simulink model "SkywalkerX8_Lateral_Control"  (R2018a)
settings: Solver=FixedStepAuto  StartTime=0.0  StopTime=inf  FixedStep=0.001  RelTol=1e-3
undefined symbols (not defined in the file): SkywalkerX8
libraries: simulink_extras x1
settings Model: EnablePacing=on  Creator=David  LastModifiedBy=David

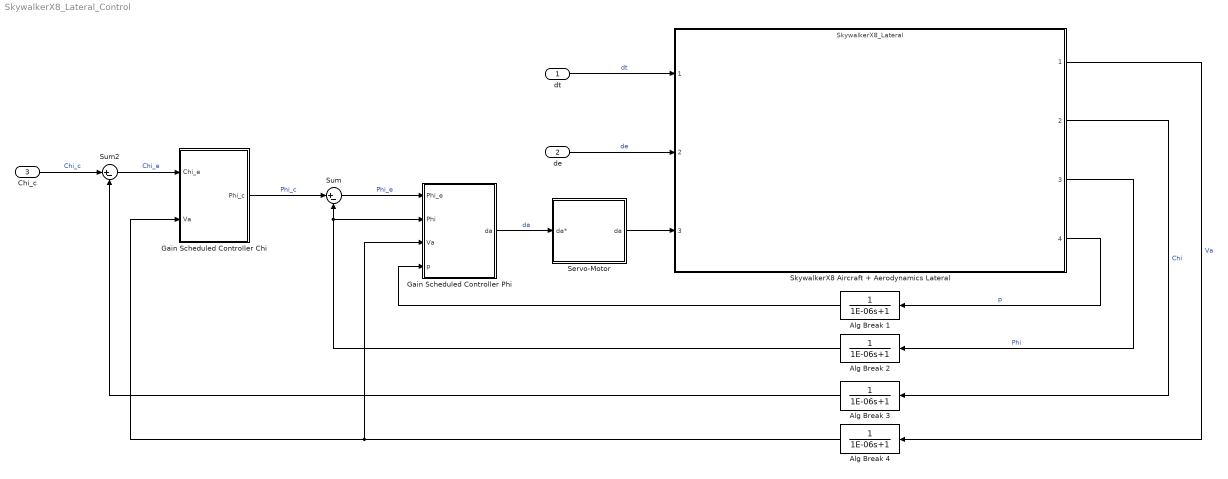
== system SkywalkerX8_Lateral_Control ==
  dt : Inport
  de : Inport  Port=2
  Chi_c : Inport  Port=3
  Alg Break {1..4} (4 alike) : TransferFcn  Denominator=[1E-06 1]
  Gain Scheduled Controller Chi : Subsystem
  Gain Scheduled Controller Phi : Subsystem
  Servo-Motor : Subsystem
      mask Display: image('servo.jpg', 'center')
  SkywalkerX8 Aircraft + Aerodynamics Lateral : ModelReference  ModelNameDialog=SkywalkerX8_Lateral.slx  ModelReferenceVersion=1.51
      mask Display:
      | image('x8SkySunset.png', 'center')
      | 
      | port_label('input', 1, '\delta_t (Unitless)', 'texmode', 'on')
      | port_label('input', 2, '\delta_e (rad)', 'texmode', 'on')
      | port_label('input', 3, '\delta_a (rad)', 'texmode', 'on')
      | 
      | port_label('output', 1, 'V_a (m/s)', 'texmode', 'on')
      | port_label('output', 2, '\chi (rad)', 'texmode', 'on')
      | port_label('output', 3, '\Phi (rad)', 'texmode', 'on')
      | port_label('output', 4, 'p (rad/s)', 'texmode', 'on')
  Sum : Sum  Inputs=|+-
  Sum2 : Sum  Inputs=|+-
  wires:
  SkywalkerX8 Aircraft + Aerodynamics Lateral/3 -> Alg Break 2/1  "Phi"
  SkywalkerX8 Aircraft + Aerodynamics Lateral/1 -> Alg Break 4/1  "Va"
  SkywalkerX8 Aircraft + Aerodynamics Lateral/2 -> Alg Break 3/1  "Chi"
  Gain Scheduled Controller Chi/1(Phi_c) -> Sum/1  "Phi_c"
  Chi_c/1 -> Sum2/1  "Chi_c"
  Sum/1 -> Gain Scheduled Controller Phi/1(Phi_e)  "Phi_e"
  Sum2/1 -> Gain Scheduled Controller Chi/1(Chi_e)  "Chi_e"
  Alg Break 4/1 -> Gain Scheduled Controller Chi/2(Va), Gain Scheduled Controller Phi/3(Va)
  Alg Break 2/1 -> Gain Scheduled Controller Phi/2(Phi), Sum/2
  Gain Scheduled Controller Phi/1(da) -> Servo-Motor/1(da*)  "da"
  Alg Break 1/1 -> Gain Scheduled Controller Phi/4(p)
  de/1 -> SkywalkerX8 Aircraft + Aerodynamics Lateral/2  "de"
  dt/1 -> SkywalkerX8 Aircraft + Aerodynamics Lateral/1  "dt"
  SkywalkerX8 Aircraft + Aerodynamics Lateral/4 -> Alg Break 1/1  "p"
  Alg Break 3/1 -> Sum2/2
  Servo-Motor/1(da) -> SkywalkerX8 Aircraft + Aerodynamics Lateral/3

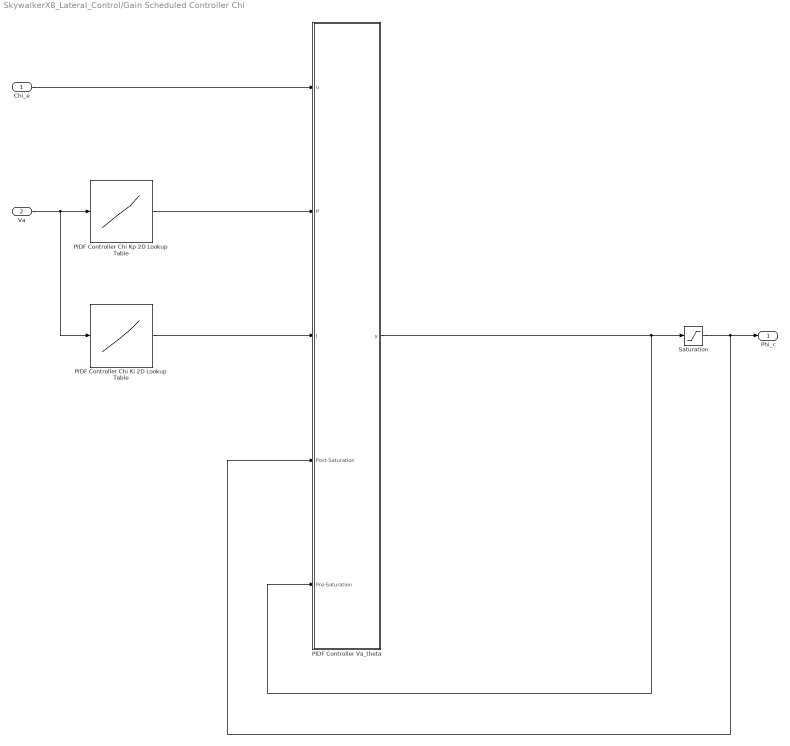
== system SkywalkerX8_Lateral_Control/Gain Scheduled Controller Chi ==
  Chi_e : Inport
  Va : Inport  Port=2
  PIDF Controller Chi Ki 2D Lookup Table : Lookup_n-D  NumberOfTableDimensions=1  BreakpointsForDimension1=SkywalkerX8.Control.Lateral.SchedulingVariables.VaArray  BreakpointsForDimension2=SkywalkerX8.Control.Longitudinal.SchedulingVariables.alphaArray  Table=SkywalkerX8.Control.Lateral.ChiController.KiChi  InternalRulePriority=Speed  RndMeth=Simplest  InputSameDT=on
  PIDF Controller Chi Kp 2D Lookup Table : Lookup_n-D  NumberOfTableDimensions=1  BreakpointsForDimension1=SkywalkerX8.Control.Lateral.SchedulingVariables.VaArray  BreakpointsForDimension2=SkywalkerX8.Control.Longitudinal.SchedulingVariables.alphaArray  Table=SkywalkerX8.Control.Lateral.ChiController.KpChi  InternalRulePriority=Speed  RndMeth=Simplest  InputSameDT=on
  PIDF Controller Va_theta : Subsystem
  Saturation : Saturate  UpperLimit=SkywalkerX8.Control.Lateral.ChiController.upperSaturationPhiC  LowerLimit=SkywalkerX8.Control.Lateral.ChiController.lowerSaturationPhiC
  Phi_c : Outport
  wires:
  PIDF Controller Chi Kp 2D Lookup Table/1 -> PIDF Controller Va_theta/2(P)
  Chi_e/1 -> PIDF Controller Va_theta/1(u)
  Va/1 -> PIDF Controller Chi Ki 2D Lookup Table/1, PIDF Controller Chi Kp 2D Lookup Table/1
  PIDF Controller Chi Ki 2D Lookup Table/1 -> PIDF Controller Va_theta/3(I)
  Saturation/1 -> PIDF Controller Va_theta/4(Post-Saturation), Phi_c/1
  PIDF Controller Va_theta/1(y) -> PIDF Controller Va_theta/5(Pre-Saturation), Saturation/1

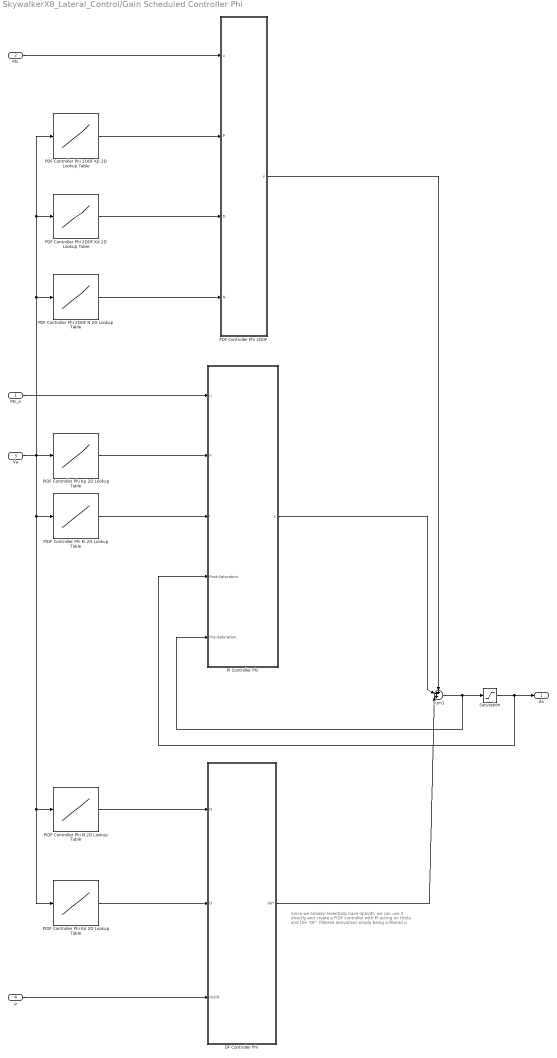
== system SkywalkerX8_Lateral_Control/Gain Scheduled Controller Phi ==
  note: Since we already essentially have dphi/dt,
      | we can use it directly and create a PIDF controller
      | with PI acting on theta and the "DF" (filtered derivative)
      | simply being a filtered p
  Phi_e : Inport
  Phi : Inport  Port=2
  Va : Inport  Port=3
  p : Inport  Port=4
  DF Controller Phi : Subsystem
  PDF Controller Phi 2DOF : Subsystem
  PDF Controller Phi 2DOF Kd 2D Lookup Table : Lookup_n-D  NumberOfTableDimensions=1  BreakpointsForDimension1=SkywalkerX8.Control.Lateral.SchedulingVariables.VaArray  BreakpointsForDimension2=SkywalkerX8.Control.Longitudinal.SchedulingVariables.alphaArray  Table=SkywalkerX8.Control.Lateral.PhiController.KdPhi2DOF  InternalRulePriority=Speed  RndMeth=Simplest  InputSameDT=on
  PDF Controller Phi 2DOF Kp 2D Lookup Table : Lookup_n-D  NumberOfTableDimensions=1  BreakpointsForDimension1=SkywalkerX8.Control.Lateral.SchedulingVariables.VaArray  BreakpointsForDimension2=SkywalkerX8.Control.Longitudinal.SchedulingVariables.alphaArray  Table=SkywalkerX8.Control.Lateral.PhiController.KpPhi2DOF  InternalRulePriority=Speed  RndMeth=Simplest  InputSameDT=on
  PDF Controller Phi 2DOF N 2D Lookup Table : Lookup_n-D  NumberOfTableDimensions=1  BreakpointsForDimension1=SkywalkerX8.Control.Lateral.SchedulingVariables.VaArray  BreakpointsForDimension2=SkywalkerX8.Control.Longitudinal.SchedulingVariables.alphaArray  Table=SkywalkerX8.Control.Lateral.PhiController.NPhi2DOF  InternalRulePriority=Speed  RndMeth=Simplest  InputSameDT=on
  PI Controller Phi : Subsystem
  PIDF Controller Phi Kd 2D Lookup Table : Lookup_n-D  NumberOfTableDimensions=1  BreakpointsForDimension1=SkywalkerX8.Control.Lateral.SchedulingVariables.VaArray  BreakpointsForDimension2=SkywalkerX8.Control.Longitudinal.SchedulingVariables.alphaArray  Table=SkywalkerX8.Control.Lateral.PhiController.KdPhi  InternalRulePriority=Speed  RndMeth=Simplest  InputSameDT=on
  PIDF Controller Phi Ki 2D Lookup Table : Lookup_n-D  NumberOfTableDimensions=1  BreakpointsForDimension1=SkywalkerX8.Control.Lateral.SchedulingVariables.VaArray  BreakpointsForDimension2=SkywalkerX8.Control.Longitudinal.SchedulingVariables.alphaArray  Table=SkywalkerX8.Control.Lateral.PhiController.KiPhi  InternalRulePriority=Speed  RndMeth=Simplest  InputSameDT=on
  PIDF Controller Phi Kp 2D Lookup Table : Lookup_n-D  NumberOfTableDimensions=1  BreakpointsForDimension1=SkywalkerX8.Control.Lateral.SchedulingVariables.VaArray  BreakpointsForDimension2=SkywalkerX8.Control.Longitudinal.SchedulingVariables.alphaArray  Table=SkywalkerX8.Control.Lateral.PhiController.KpPhi  InternalRulePriority=Speed  RndMeth=Simplest  InputSameDT=on
  PIDF Controller Phi N 2D Lookup Table : Lookup_n-D  NumberOfTableDimensions=1  BreakpointsForDimension1=SkywalkerX8.Control.Lateral.SchedulingVariables.VaArray  BreakpointsForDimension2=SkywalkerX8.Control.Longitudinal.SchedulingVariables.alphaArray  Table=SkywalkerX8.Control.Lateral.PhiController.NPhi  InternalRulePriority=Speed  RndMeth=Simplest  InputSameDT=on
  Saturation : Saturate  UpperLimit=SkywalkerX8.Control.Lateral.PhiController.upperSaturationDa  LowerLimit=SkywalkerX8.Control.Lateral.PhiController.lowerSaturationDa
  Sum1 : Sum  Inputs=+++|
  da : Outport
  wires:
  Va/1 -> PDF Controller Phi 2DOF Kp 2D Lookup Table/1, PDF Controller Phi 2DOF Kd 2D Lookup Table/1, PDF Controller Phi 2DOF N 2D Lookup Table/1, PIDF Controller Phi N 2D Lookup Table/1, PIDF Controller Phi Kd 2D Lookup Table/1, PIDF Controller Phi Ki 2D Lookup Table/1, PIDF Controller Phi Kp 2D Lookup Table/1
  Phi_e/1 -> PI Controller Phi/1(u)
  PIDF Controller Phi Kp 2D Lookup Table/1 -> PI Controller Phi/2(P)
  PIDF Controller Phi Ki 2D Lookup Table/1 -> PI Controller Phi/3(I)
  PI Controller Phi/1(y) -> Sum1/2
  Sum1/1 -> Saturation/1, PI Controller Phi/5(Pre-Saturation)
  p/1 -> DF Controller Phi/3(du/dt)
  DF Controller Phi/1(da*) -> Sum1/3
  PIDF Controller Phi N 2D Lookup Table/1 -> DF Controller Phi/1(N)
  PIDF Controller Phi Kd 2D Lookup Table/1 -> DF Controller Phi/2(D)
  Saturation/1 -> da/1, PI Controller Phi/4(Post-Saturation)
  PDF Controller Phi 2DOF Kp 2D Lookup Table/1 -> PDF Controller Phi 2DOF/2(P)
  PDF Controller Phi 2DOF Kd 2D Lookup Table/1 -> PDF Controller Phi 2DOF/3(D)
  PDF Controller Phi 2DOF N 2D Lookup Table/1 -> PDF Controller Phi 2DOF/4(N)
  Phi/1 -> PDF Controller Phi 2DOF/1(u)
  PDF Controller Phi 2DOF/1(y) -> Sum1/1

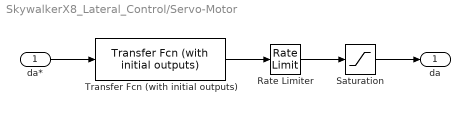
== system SkywalkerX8_Lateral_Control/Servo-Motor ==
  da* : Inport
  Rate Limiter : RateLimiter  RisingSlewLimit=SkywalkerX8.Actuators.Servos.RateLimit  FallingSlewLimit=-SkywalkerX8.Actuators.Servos.RateLimit  SampleTimeMode=inherited  InitialCondition=SkywalkerX8.InitialConditions.de
  Saturation : Saturate  UpperLimit=2*SkywalkerX8.Actuators.Servos.UpperSaturation  LowerLimit=2*SkywalkerX8.Actuators.Servos.LowerSaturation
  Transfer Fcn (with initial outputs) : simulink_extras/Additional Linear/Transfer Fcn (with initial outputs)  N=cell2mat(SkywalkerX8.Actuators.Servos.TF.Numerator)  D=cell2mat(SkywalkerX8.Actuators.Servos.TF.Denominator)  Y0=SkywalkerX8.InitialConditions.da  U0=SkywalkerX8.InitialConditions.da
  da : Outport
  wires:
  Rate Limiter/1 -> Saturation/1
  da*/1 -> Transfer Fcn (with initial outputs)/1
  Saturation/1 -> da/1
  Transfer Fcn (with initial outputs)/1 -> Rate Limiter/1

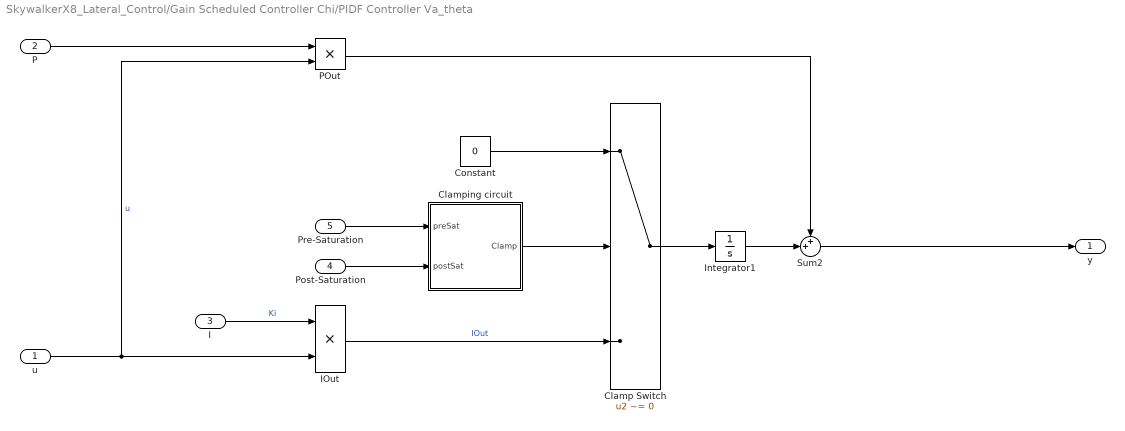
== system SkywalkerX8_Lateral_Control/Gain Scheduled Controller Chi/PIDF Controller Va_theta ==
  u : Inport
  P : Inport  Port=2
  I : Inport  Port=3
  Post-Saturation : Inport  Port=4
  Pre-Saturation : Inport  Port=5
  Clamp Switch : Switch  Criteria=u2 ~= 0
  Clamping circuit : Subsystem
  Constant : Constant  Value=0
  IOut : Product  DisableCoverage=on
  Integrator1 : Integrator  IgnoreLimit=on
  POut : Product
  Sum2 : Sum  Inputs=++|
  y : Outport  InitialOutput=0
  wires:
  Sum2/1 -> y/1
  POut/1 -> Sum2/1
  u/1 -> POut/2, IOut/2  "u"
  Clamp Switch/1 -> Integrator1/1
  Integrator1/1 -> Sum2/2
  Constant/1 -> Clamp Switch/1
  I/1 -> IOut/1  "Ki"
  IOut/1 -> Clamp Switch/3  "IOut"
  Clamping circuit/1(Clamp) -> Clamp Switch/2
  P/1 -> POut/1
  Pre-Saturation/1 -> Clamping circuit/1(preSat)
  Post-Saturation/1 -> Clamping circuit/2(postSat)

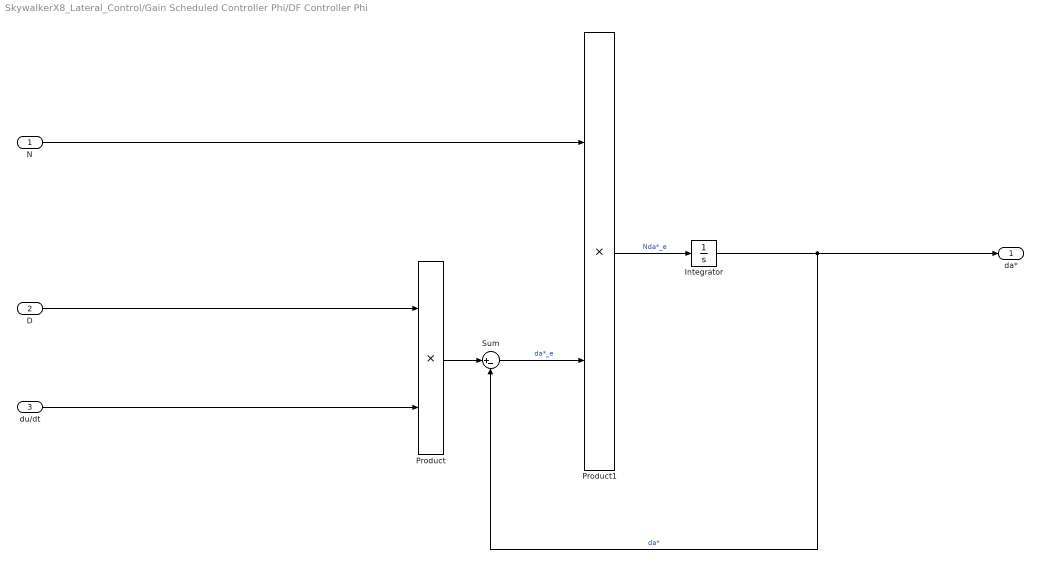
== system SkywalkerX8_Lateral_Control/Gain Scheduled Controller Phi/DF Controller Phi ==
  N : Inport
  D : Inport  Port=2
  du/dt : Inport  Port=3
  Integrator : Integrator
  Product : Product
  Product1 : Product
  Sum : Sum  Inputs=|+-
  da* : Outport
  wires:
  Integrator/1 -> da*/1, Sum/2  "da*"
  Product1/1 -> Integrator/1  "Nda*_e"
  du/dt/1 -> Product/2
  D/1 -> Product/1
  Sum/1 -> Product1/2  "da*_e"
  N/1 -> Product1/1
  Product/1 -> Sum/1

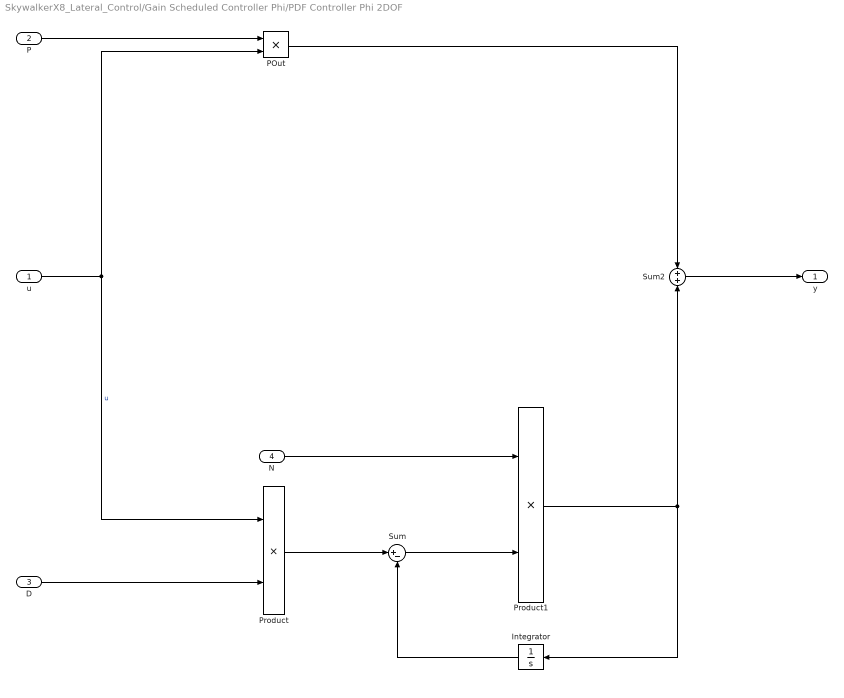
== system SkywalkerX8_Lateral_Control/Gain Scheduled Controller Phi/PDF Controller Phi 2DOF ==
  u : Inport
  P : Inport  Port=2
  D : Inport  Port=3
  N : Inport  Port=4
  Integrator : Integrator
  POut : Product
  Product : Product
  Product1 : Product
  Sum : Sum  Inputs=|+-
  Sum2 : Sum
  y : Outport  InitialOutput=0
  wires:
  Sum2/1 -> y/1
  N/1 -> Product1/1
  Product1/1 -> Sum2/2, Integrator/1
  Sum/1 -> Product1/2
  POut/1 -> Sum2/1
  D/1 -> Product/2
  u/1 -> Product/1, POut/2  "u"
  Integrator/1 -> Sum/2
  Product/1 -> Sum/1
  P/1 -> POut/1

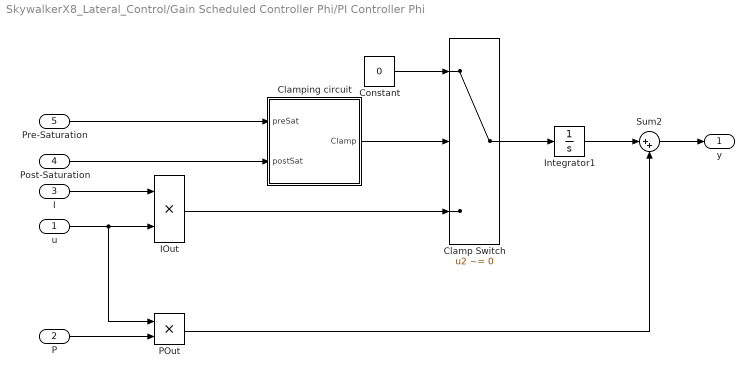
== system SkywalkerX8_Lateral_Control/Gain Scheduled Controller Phi/PI Controller Phi ==
  u : Inport
  P : Inport  Port=2
  I : Inport  Port=3
  Post-Saturation : Inport  Port=4
  Pre-Saturation : Inport  Port=5
  Clamp Switch : Switch  Criteria=u2 ~= 0
  Clamping circuit : Subsystem
  Constant : Constant  Value=0
  IOut : Product  DisableCoverage=on
  Integrator1 : Integrator  InitialCondition=SkywalkerX8.InitialConditions.da  IgnoreLimit=on
  POut : Product
  Sum2 : Sum  Inputs=|++
  y : Outport  InitialOutput=0
  wires:
  IOut/1 -> Clamp Switch/3
  Clamp Switch/1 -> Integrator1/1
  Sum2/1 -> y/1
  Pre-Saturation/1 -> Clamping circuit/1(preSat)
  Post-Saturation/1 -> Clamping circuit/2(postSat)
  Clamping circuit/1(Clamp) -> Clamp Switch/2
  Constant/1 -> Clamp Switch/1
  Integrator1/1 -> Sum2/1
  POut/1 -> Sum2/2
  P/1 -> POut/2
  u/1 -> POut/1, IOut/2
  I/1 -> IOut/1

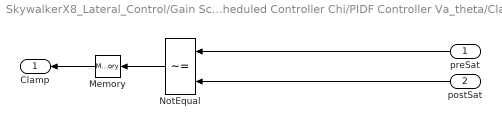
== system SkywalkerX8_Lateral_Control/Gain Scheduled Controller Chi/PIDF Controller Va_theta/Clamping circuit ==
  preSat : Inport  DisableCoverage=on
  postSat : Inport  DisableCoverage=on  Port=2
  Memory : Memory  DisableCoverage=on
  NotEqual : RelationalOperator  DisableCoverage=on  Operator=~=  RndMeth=Nearest  InputSameDT=on
  Clamp : Outport  DisableCoverage=on
  wires:
  postSat/1 -> NotEqual/2
  preSat/1 -> NotEqual/1
  NotEqual/1 -> Memory/1
  Memory/1 -> Clamp/1

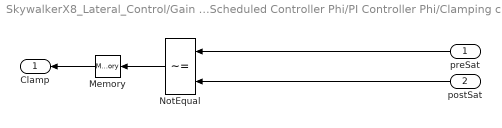
== system SkywalkerX8_Lateral_Control/Gain Scheduled Controller Phi/PI Controller Phi/Clamping circuit ==
  preSat : Inport  DisableCoverage=on
  postSat : Inport  DisableCoverage=on  Port=2
  Memory : Memory  DisableCoverage=on
  NotEqual : RelationalOperator  DisableCoverage=on  Operator=~=  RndMeth=Nearest  InputSameDT=on
  Clamp : Outport  DisableCoverage=on
  wires:
  postSat/1 -> NotEqual/2
  preSat/1 -> NotEqual/1
  NotEqual/1 -> Memory/1
  Memory/1 -> Clamp/1
